simulink model "sgMdl_IO672_MILSTD1553Loopback"  (R2024b)
settings: Solver=FixedStepAuto  StartTime=0.0  StopTime=inf  RelTol=1e-3  EnableMultiTasking=on
undefined symbols (not defined in the file): IO672, MF, SF
libraries: speedgoatlib_IO672 x11, slrealtimeutilitieslib x4
Description:
  | IO672 - MIL-STD-1553 Loopback
settings Model: sg_rtwmakecfg_data=_mil-std-1553__ge_1553_  ModifiedByFormat=Speedgoat  Creator=Speedgoat  LastModifiedBy=Speedgoat
settings SolverCC: ConcurrentTasks=on  AlgebraicLoopSolver=TrustRegion  PositivePriorityOrder=on
settings DataIOCC: LimitDataPoints=on  SaveFormat=Array  ReturnWorkspaceOutputs=off
settings OptimizationCC: BlockReduction=off  OptimizeBlockIOStorage=off  BufferReuse=off  ReuseModelBlockBuffer=off  GlobalBufferReuse=off  ExpressionFolding=off  LocalBlockOutputs=off  OptimizeDataStoreBuffers=off  BusAssignmentInplaceUpdate=off
settings DebuggingCC: SolverPrmCheckMsg=warning  TasksWithSamePriorityMsg=none  UnconnectedInputMsg=warning  UnconnectedOutputMsg=warning  UnconnectedLineMsg=warning  AllowSymbolicDim=off  SFUnexpectedBacktrackingDiag=warning  SFNoUnconditionalDefaultTransitionDiag=warning  SFExecutionAtInitializationDiag=none  ArithmeticOperatorsInVariantConditions=warning
settings HardwareCC: ProdBitPerLong=64  ProdLongLongMode=on  ProdHWDeviceType=Intel->x86-64 (Linux 64)
settings ModelReferenceCC: EnableRefExpFcnMdlSchedulingChecks=on  PropagateSignalLabelsOutOfModel=off
settings SFSimCC: SimUseLocalCustomCode=off  CustomCodeUndefinedFunction=UseInterfaceOnly
settings RTWCC: Description=Speedgoat Real-Time Target Machine  SystemTargetFile=speedgoat.tlc  TemplateMakefile=slrealtime_default_tmf  RTWUseLocalCustomCode=off  Toolchain=Simulink Real-Time Toolchain  BuildConfiguration=Faster Runs  TargetLang=C++  GPUComputeCapability=3.5  DLArmComputeVersion=19.05
settings CodeAppCC: StateflowObjectComments=on
settings SimulinkRealTimeTargetCC: SubcomponentCodeInterfacePackaging=Reusable function  InstructionSetFMA=off  LogToMDFFile=off  SLRTFileLogMaxRuns=10  UseGCCFastMath=on
settings ConfigComp: CovMetricSettings=dw  CovSaveCumulativeToWorkspaceVar=on  CovSaveSingleToWorkspaceVar=on  CovExternalEMLEnable=off  CovSFcnEnable=off  CovBoundaryAbsTol=1.0e-5

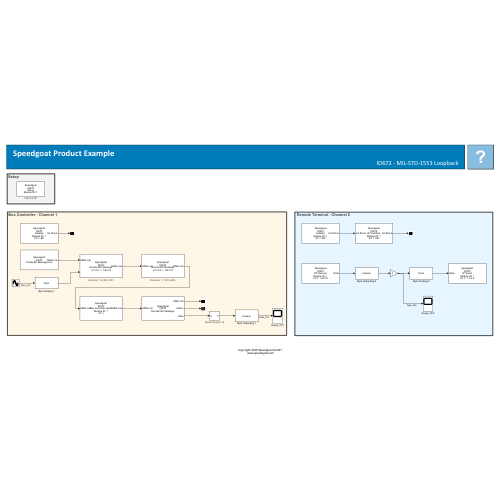
[thumbnail: Simulink's stored preview of the top-level diagram]
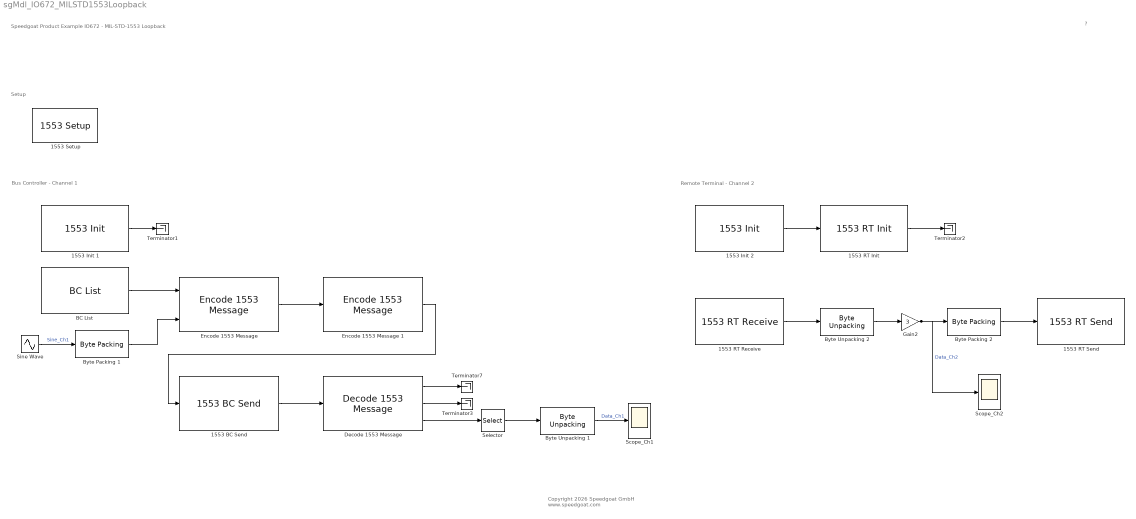
== system sgMdl_IO672_MILSTD1553Loopback ==
  note: Setup
  note: Bus Controller - Channel 1
  note: Remote Terminal - Channel 2
  note: Speedgoat Product Example
      | IO672 - MIL-STD-1553 Loopback
  note: ?
  note: Copyright 2026 Speedgoat GmbH
      |  www.speedgoat.com
  1553 BC Send : speedgoatlib_IO672/1553 BC Send  id=1  channel=1  waitflag=Send new message then wait and read response  waittime=1000  sampletime=-1  slot=-1  boardtype=IO672-4-MF
      settings: SourceProductName=Simulink Real-Time: Speedgoat I/O Blockset
  1553 Init 1 : speedgoatlib_IO672/1553 Init   id=1  boardtype=IO672-4-MF  channel=1  loopback=off  coupling=Direct Coupling  voltage=5.0  initbc=on  nbcbuffs=2  retryenabled=off  nrtimeout=14  lrtimeout=12  initbm=off  mona=on  monb=off  nbmbuffs=100  initrt=off  broadcast=off  sampleTime=0.01  slot=-1
      settings: SourceProductName=Simulink Real-Time: Speedgoat I/O Blockset
  1553 Init 2 : speedgoatlib_IO672/1553 Init   id=1  boardtype=IO672-4-MF  channel=2  loopback=off  coupling=Direct Coupling  voltage=5.0  initbc=off  nbcbuffs=5  retryenabled=off  nrtimeout=14  lrtimeout=12  initbm=off  mona=on  monb=off  nbmbuffs=100  initrt=on  broadcast=off  sampleTime=0.01  slot=-1
      settings: SourceProductName=Simulink Real-Time: Speedgoat I/O Blockset
  "1553 RT Init " : speedgoatlib_IO672/1553 RT Init   id=1  rt=1  enableA=on  enableB=on  status=0  bit=0  itf=off  tsubs=[0 3]  tlengths=[hex2dec('FFFFFFFF') hex2dec('FFFFFFFF')]  rsubs=[0 3]  rlengths=[hex2dec('FFFFFFFF') hex2dec('FFFFFFFF')]  sampleTime=-1  parEnBusA=off  parEnBusB=off  boardtype=IO672-4-MF
      settings: SourceProductName=Simulink Real-Time: Speedgoat I/O Blockset
  "1553 RT Receive " : speedgoatlib_IO672/1553 RT Receive   id=1  channel=2  rt=1  sub=3  reccount=4  timestamp=off  sampleTime=0.01  slot=-1  boardtype=IO672-4-MF
      settings: SourceProductName=Simulink Real-Time: Speedgoat I/O Blockset
  "1553 RT Send " : speedgoatlib_IO672/1553 RT Send   id=1  channel=2  rt=1  sub=3  sendcount=4  sampleTime=-1  slot=-1  boardtype=IO672-4-MF
      settings: SourceProductName=Simulink Real-Time: Speedgoat I/O Blockset
  1553 Setup : speedgoatlib_IO672/1553 Setup  id=1  boardtype=IO672-2-SF  slot=-1
      settings: AttributesFormatString=%<boardtype>  SourceProductName=Simulink Real-Time: Speedgoat I/O Blockset
  "BC List " : speedgoatlib_IO672/Utilities/BC List   num=2  sampletime=0.01
      settings: SourceProductName=Simulink Real-Time: Speedgoat I/O Blockset
  Byte Packing 1 : slrealtimeutilitieslib/Byte Packing  MaskPackedDataType=uint16  MaskUnpackedDataTypes={'double'}  MaskAlignment=1
  Byte Packing 2 : slrealtimeutilitieslib/Byte Packing  MaskPackedDataType=uint16  MaskUnpackedDataTypes={'double'}  MaskAlignment=1
  Byte Unpacking 1 : slrealtimeutilitieslib/Byte Unpacking  MaskUnpackedDataTypes={'double'}  MaskUnpackedDataSizes={[1]}  MaskAlignment=1
  Byte Unpacking 2 : slrealtimeutilitieslib/Byte Unpacking  MaskUnpackedDataTypes={'double'}  MaskUnpackedDataSizes={[1]}  MaskAlignment=1
  "Decode 1553 Message " : speedgoatlib_IO672/Utilities/Decode 1553 Message   messno=2  sampletime=-1
      settings: SourceProductName=Simulink Real-Time: Speedgoat I/O Blockset
  "Encode 1553 Message " : speedgoatlib_IO672/Utilities/Encode 1553 Message   messno=1  termaddr1=1  subaddr1=3  termaddr2=2  subaddr2=4  mode=1 Synchronize  sendcount=4  direction=R (BC->RT)  gap=30  bus=A  sampletime=-1
      settings: AttributesFormatString=Direction = %<direction>  SourceProductName=Simulink Real-Time: Speedgoat I/O Blockset
  Encode 1553 Message 1 : speedgoatlib_IO672/Utilities/Encode 1553 Message   messno=2  termaddr1=1  subaddr1=3  termaddr2=2  subaddr2=4  mode=1 Synchronize  sendcount=4  direction=T (RT->BC)  gap=10  bus=A  sampletime=-1
      settings: AttributesFormatString=Direction = %<direction>  SourceProductName=Simulink Real-Time: Speedgoat I/O Blockset
  Gain2 : Gain  Gain=3
  Scope_Ch1 : Scope
  Scope_Ch2 : Scope
  Selector : Selector  InputPortWidth=32  IndexOptions=Index vector (dialog)  Indices=[1:4]  OutputSizes=1
      settings: AttributesFormatString=Extract Bytes %<Indices>
  Sine Wave : Sin  Amplitude=10  Frequency=2*pi  SampleTime=0.01
  Terminator{1..3,7} (4 alike) : Terminator
  wires:
  "Decode 1553 Message "/1 -> Terminator7/1
  "Encode 1553 Message "/1 -> Encode 1553 Message 1/1
  1553 Init 1/1 -> Terminator1/1
  1553 BC Send/1 -> "Decode 1553 Message "/1
  "1553 RT Init "/1 -> Terminator2/1
  "BC List "/1 -> "Encode 1553 Message "/1
  1553 Init 2/1 -> "1553 RT Init "/1
  Encode 1553 Message 1/1 -> 1553 BC Send/1
  "Decode 1553 Message "/2 -> Terminator3/1
  "1553 RT Receive "/1 -> Byte Unpacking 2/1
  Sine Wave/1 -> Byte Packing 1/1  "Sine_Ch1"
  Byte Packing 1/1 -> "Encode 1553 Message "/2
  Byte Unpacking 1/1 -> Scope_Ch1/1  "Data_Ch1"
  Selector/1 -> Byte Unpacking 1/1
  "Decode 1553 Message "/3 -> Selector/1
  Byte Unpacking 2/1 -> Gain2/1
  Byte Packing 2/1 -> "1553 RT Send "/1
  Gain2/1 -> Scope_Ch2/1, Byte Packing 2/1  "Data_Ch2"
